simulink model "D_framewiseincremental_simple_vs_cascaded"  (R2017a)
settings: Solver=ode45  StartTime=0.0  StopTime=200  FixedStep=0.05  RelTol=1e-3  EnableMultiTasking=on
values from neighbouring files (symbols this model uses):
  B = [1 0.5 -0.5 -1 0 0.5 ; 0 0 0 0 2 0 ; -0.05 -0.02 0.02 0.05 0 2 ; -1 -1 -1 -1 -2 0]    [A_runSimulation.m]    (also in C_runSimulation.m; D_runSimulation.m; E_runSimulation.m; F_runSimulation.m)
  gain_four = rand()*2    [A_runSimulation.m]    (also in C_runSimulation.m = 0; D_runSimulation.m; E_runSimulation.m = 0; F_runSimulation.m = 0)
  gain_one = rand()*2    [A_runSimulation.m]    (also in C_runSimulation.m = 0; D_runSimulation.m; E_runSimulation.m = 0; F_runSimulation.m = 0)
  gain_three = rand()*2    [A_runSimulation.m]    (also in C_runSimulation.m = 0; D_runSimulation.m; E_runSimulation.m = 0; F_runSimulation.m = 0)
  gain_two = rand()*2    [A_runSimulation.m]    (also in C_runSimulation.m = 0; D_runSimulation.m; E_runSimulation.m = 0; F_runSimulation.m = 0)
  reduction_type = 1    [A_runSimulation.m]    (also in C_runSimulation.m = 2; D_runSimulation.m; E_runSimulation.m = 2)
  seed_four = k + 30    [A_runSimulation.m]    (also in C_runSimulation.m; D_runSimulation.m; E_runSimulation.m; F_runSimulation.m)
  seed_one = k    [A_runSimulation.m]    (also in C_runSimulation.m; D_runSimulation.m; E_runSimulation.m; F_runSimulation.m)
  seed_three = k + 20    [A_runSimulation.m]    (also in C_runSimulation.m; D_runSimulation.m; E_runSimulation.m; F_runSimulation.m)
  seed_two = k + 10    [A_runSimulation.m]    (also in C_runSimulation.m; D_runSimulation.m; E_runSimulation.m; F_runSimulation.m)
  signal_gain = j    [A_runSimulation.m]    (also in C_runSimulation.m; D_runSimulation.m; E_runSimulation.m = 0.3; F_runSimulation.m)
  simulate_envelope = 1    [A_runSimulation.m]    (also in C_runSimulation.m = 0; D_runSimulation.m; E_runSimulation.m = 0)
  u_lim = [[-0.5 -0.5 -0.5 -0.5 -0.5 -0.5]' [0.5 0.5 0.5 0.5 0.5 0.5]']    [A_runSimulation.m]    (also in C_runSimulation.m; D_runSimulation.m; E_runSimulation.m; F_runSimulation.m)
  udot_lim = [[2 2 2 2 2 2]']    [A_runSimulation.m]    (also in C_runSimulation.m; D_runSimulation.m; E_runSimulation.m; F_runSimulation.m)
  W = eye(6)    [A_runSimulation.m]    (also in C_runSimulation.m; D_runSimulation.m; E_runSimulation.m; F_runSimulation.m)
libraries: dspsrcs4 x8
settings Model: Creator=markvoskuijl  LastModifiedBy=Luca
settings DataIOCC: LimitDataPoints=on  SaveFormat=Array  SignalLoggingSaveFormat=ModelDataLogs
settings OptimizationCC: ExpressionDepthLimit=2147483647  LifeSpan=inf
settings DebuggingCC: UnderspecifiedInitializationDetection=Classic  MergeDetectMultiDrivingBlocksExec=none  SolverPrmCheckMsg=warning  FcnCallInpInsideContextMsg=warning  StateNameClashWarn=warning  SFUnexpectedBacktrackingDiag=warning  SFNoUnconditionalDefaultTransitionDiag=warning  SFExecutionAtInitializationDiag=none
settings HardwareCC: ProdBitPerPointer=32  ProdBitPerSizeT=32  ProdBitPerPtrDiffT=32  ProdLargestAtomicFloat=None  ProdIntDivRoundTo=Undefined  ProdEndianess=Unspecified  ProdWordSize=32  ProdHWDeviceType=32-bit Generic
settings ModelReferenceCC: PropagateSignalLabelsOutOfModel=off
settings GRTTargetCC: TargetLangStandard=C89/C90 (ANSI)  GeneratePreprocessorConditionals=Disable all  CombineOutputUpdateFcns=off  GRTInterface=on
settings ConfigComp: CovMetricSettings=dw  CovHtmlReporting=on  CovSaveCumulativeToWorkspaceVar=on  CovSaveSingleToWorkspaceVar=on  CovExternalEMLEnable=off

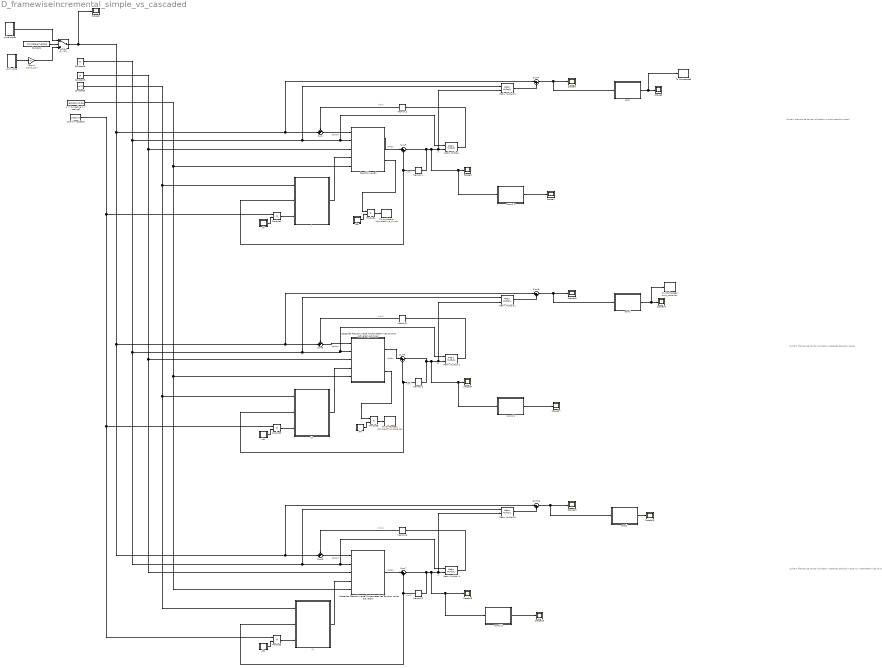
== system D_framewiseincremental_simple_vs_cascaded ==
  note: deltam
  note: deltau
  note: ut
  note: u(t-1)
  note: m(t-1)
  note: durham
      | (framewise control allocation
      | simple pseudoinverse)
  note: deltam
  note: u(t-1)
  note: m(t-1)
  note: ut
  note: durham
      | (framewise control allocation
      | cascaded pseudoinverse
      | no underdetermined solution)
  note: deltau
  note: m(t-1)
  note: deltam
  note: u(t-1)
  note: ut
  note: deltau
  note: durham
      | (framewise control allocation
      | cascaded pseudoinverse)
  "1 -> truncating 2 -> scaling1" : Constant  Value=reduction_type
  Cascaded Pseudoinverse (Under deterined solution never activated) : MATLAB Function  TreatAsAtomicUnit=on
  Cascaded Pseudoinverse (Under determined solution activated just once) : MATLAB Function  TreatAsAtomicUnit=on
  Constant : Constant  Value=simulate_envelope
  Constant4 : Constant  Value=u_lim
  Constant5 : Constant  Value=W
  Constant6 : Constant  Value=B
  Gain4 : Gain  Gain=signal_gain
  I : MATLAB Function  TreatAsAtomicUnit=on
  I1 : MATLAB Function  TreatAsAtomicUnit=on
  I3 : MATLAB Function  TreatAsAtomicUnit=on
  Matrix Multiply{,1..5} (6 alike) : Product  Multiplication=Matrix(*)
  Memory{1..6} (6 alike) : Memory
  Product{1..5} (5 alike) : Product
  Pseudoinverse1 : MATLAB Function  TreatAsAtomicUnit=on
  Scope{1..3,5..6,13..15,19,24..27} (13 alike) : Scope
  Sum : Sum  Inputs=-+|
  Sum10 : Sum  Inputs=|-+
  Sum3 : Sum  Inputs=|++
  Sum4 : Sum  Inputs=|-+
  Sum5 : Sum  Inputs=-+|
  Sum6 : Sum  Inputs=-+|
  Sum7 : Sum  Inputs=|++
  Sum8 : Sum  Inputs=|++
  Sum9 : Sum  Inputs=|-+
  Switch : Switch  Threshold=1
  To Workspace : ToWorkspace  VariableName=saturatedtime_simple  SampleTime=-1
      settings: Save2DSignal=2-D array (concatenate along first dimension)
  To Workspace1 : ToWorkspace  VariableName=saturatedtime_cascaded  SampleTime=-1
      settings: Save2DSignal=2-D array (concatenate along first dimension)
  To Workspace2 : ToWorkspace  VariableName=error_cascaded  SampleTime=-1
      settings: Save2DSignal=2-D array (concatenate along first dimension)
  To Workspace3 : ToWorkspace  VariableName=error_simple  SampleTime=-1
      settings: Save2DSignal=2-D array (concatenate along first dimension)
  dt : Subsystem
  dt1 : Subsystem
  dt2 : Subsystem
  dt3 : Subsystem
  dt4 : Subsystem
  error : MATLAB Function  TreatAsAtomicUnit=on
  error1 : MATLAB Function  TreatAsAtomicUnit=on
  error2 : MATLAB Function  TreatAsAtomicUnit=on
  norm2 1 : MATLAB Function  TreatAsAtomicUnit=on
  norm2 2 : MATLAB Function  TreatAsAtomicUnit=on
  norm2 3 : MATLAB Function  TreatAsAtomicUnit=on
  pink noise : Subsystem
  udot lim rad/sec3 : Constant  Value=udot_lim
  white noise : Subsystem
  wires:
  Sum/1 -> Pseudoinverse1/1(m)
  Matrix Multiply/1 -> Memory2/1
  I/1(I) -> Pseudoinverse1/4(u_lim)
  Pseudoinverse1/1(u) -> Sum3/1
  Product1/1 -> I/3(udotdt_lim)  "udot dt"
  dt/1(dt) -> Product1/2
  Memory1/1 -> I/2(u), Sum3/2
  Memory2/1 -> Sum/1
  Matrix Multiply3/1 -> Sum4/2
  Sum4/1 -> error/1(e), Scope6/1
  Sum3/1 -> norm2 1/1(u), Scope5/1, Matrix Multiply3/2, Matrix Multiply/2, Memory1/1
  Matrix Multiply2/1 -> Sum9/2
  Sum8/1 -> norm2 2/1(u), Scope14/1, Matrix Multiply2/2, Matrix Multiply1/2, Memory3/1
  dt1/1(dt) -> Product2/2
  Memory4/1 -> Sum5/1
  Sum9/1 -> error1/1(e), Scope15/1
  Memory3/1 -> I3/2(u), Sum8/2
  Matrix Multiply1/1 -> Memory4/1
  Product2/1 -> I3/3(udotdt_lim)  "udot dt"
  Cascaded Pseudoinverse (Under determined solution activated just once)/1(u) -> Sum8/1
  Sum5/1 -> Cascaded Pseudoinverse (Under determined solution activated just once)/1(m)
  I3/1(I) -> Cascaded Pseudoinverse (Under determined solution activated just once)/4(u_lim)
  Cascaded Pseudoinverse (Under deterined solution never activated)/1(u) -> Sum7/1
  Sum6/1 -> Cascaded Pseudoinverse (Under deterined solution never activated)/1(m)
  Constant4/1 -> I/1(u_lim), I1/1(u_lim), I3/1(u_lim)
  dt2/1(dt) -> Product3/2
  Product3/1 -> I1/3(udotdt_lim)  "udot dt"
  Memory5/1 -> I1/2(u), Sum7/2
  Constant6/1 -> Matrix Multiply3/1, Matrix Multiply/1, Pseudoinverse1/2(B), Matrix Multiply5/1, Cascaded Pseudoinverse (Under deterined solution never activated)/2(B), Matrix Multiply4/1, Matrix Multiply2/1, Cascaded Pseudoinverse (Under determined solution activated just once)/2(B), Matrix Multiply1/1
  Matrix Multiply4/1 -> Memory6/1
  Constant5/1 -> Cascaded Pseudoinverse (Under deterined solution never activated)/3(W), Cascaded Pseudoinverse (Under determined solution activated just once)/3(W), Pseudoinverse1/3(W)
  Memory6/1 -> Sum6/1
  udot lim rad/sec3/1 -> Product2/1, Product3/1, Product1/1
  "1 -> truncating 2 -> scaling1"/1 -> Pseudoinverse1/5(reductionType), Cascaded Pseudoinverse (Under deterined solution never activated)/5(reductionType), Cascaded Pseudoinverse (Under determined solution activated just once)/5(reductionType)
  Matrix Multiply5/1 -> Sum10/2
  I1/1(I) -> Cascaded Pseudoinverse (Under deterined solution never activated)/4(u_lim)
  error1/1(error) -> To Workspace2/1, Scope24/1
  Sum10/1 -> error2/1(e), Scope19/1
  Sum7/1 -> norm2 3/1(u), Scope13/1, Matrix Multiply5/2, Matrix Multiply4/2, Memory5/1
  Switch/1 -> Scope3/1, Sum4/1, Sum/2, Sum10/1, Sum6/2, Sum9/1, Sum5/2
  error/1(error) -> To Workspace3/1, Scope2/1
  error2/1(error) -> Scope25/1
  norm2 1/1(norm2) -> Scope1/1
  norm2 2/1(norm2) -> Scope27/1
  norm2 3/1(norm2) -> Scope26/1
  pink noise/1(Out1) -> Gain4/1
  Gain4/1 -> Switch/3
  Constant/1 -> Switch/2
  white noise/1(Out1) -> Switch/1
  Pseudoinverse1/2(saturated) -> Product4/1
  dt3/1(dt) -> Product4/2
  Product4/1 -> To Workspace/1
  Cascaded Pseudoinverse (Under determined solution activated just once)/2(saturated) -> Product5/1
  dt4/1(dt) -> Product5/2
  Product5/1 -> To Workspace1/1

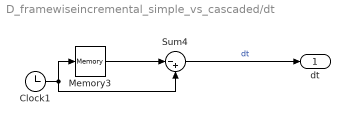
== system D_framewiseincremental_simple_vs_cascaded/dt ==
  Clock1 : Clock
  Memory3 : Memory
  Sum4 : Sum  Inputs=|-+
  dt : Outport
  wires:
  Clock1/1 -> Sum4/2, Memory3/1
  Memory3/1 -> Sum4/1
  Sum4/1 -> dt/1  "dt"

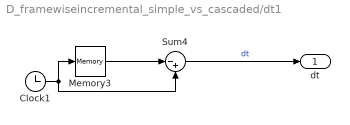
== system D_framewiseincremental_simple_vs_cascaded/dt1 ==
  Clock1 : Clock
  Memory3 : Memory
  Sum4 : Sum  Inputs=|-+
  dt : Outport
  wires:
  Clock1/1 -> Sum4/2, Memory3/1
  Memory3/1 -> Sum4/1
  Sum4/1 -> dt/1  "dt"

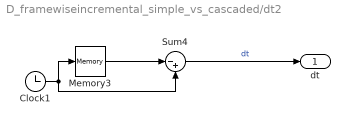
== system D_framewiseincremental_simple_vs_cascaded/dt2 ==
  Clock1 : Clock
  Memory3 : Memory
  Sum4 : Sum  Inputs=|-+
  dt : Outport
  wires:
  Clock1/1 -> Sum4/2, Memory3/1
  Memory3/1 -> Sum4/1
  Sum4/1 -> dt/1  "dt"

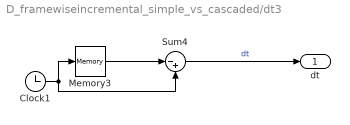
== system D_framewiseincremental_simple_vs_cascaded/dt3 ==
  Clock1 : Clock
  Memory3 : Memory
  Sum4 : Sum  Inputs=|-+
  dt : Outport
  wires:
  Clock1/1 -> Sum4/2, Memory3/1
  Memory3/1 -> Sum4/1
  Sum4/1 -> dt/1  "dt"

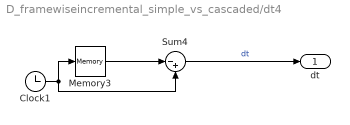
== system D_framewiseincremental_simple_vs_cascaded/dt4 ==
  Clock1 : Clock
  Memory3 : Memory
  Sum4 : Sum  Inputs=|-+
  dt : Outport
  wires:
  Clock1/1 -> Sum4/2, Memory3/1
  Memory3/1 -> Sum4/1
  Sum4/1 -> dt/1  "dt"

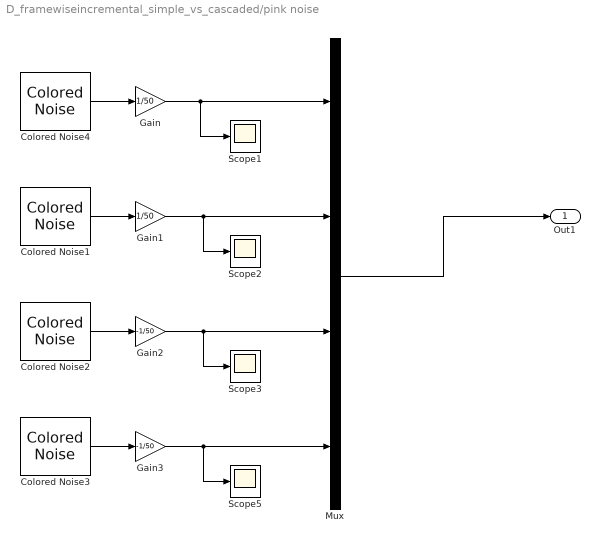
== system D_framewiseincremental_simple_vs_cascaded/pink noise ==
  Colored Noise1 : dspsrcs4/Colored Noise  Color=custom  InverseFrequencyPower=2  NumChannels=1  OutputDataType=single  SamplesPerFrame=1  SampleTime=0.1  RandomStream=mt19937ar with seed  Seed=seed_two  SimulateUsing=Interpreted execution
      settings: SourceProductName=DSP System Toolbox  SourceProductBaseCode=DS
  Colored Noise2 : dspsrcs4/Colored Noise  Color=custom  InverseFrequencyPower=2  NumChannels=1  OutputDataType=single  SamplesPerFrame=1  SampleTime=0.1  RandomStream=mt19937ar with seed  Seed=seed_three  SimulateUsing=Interpreted execution
      settings: SourceProductName=DSP System Toolbox  SourceProductBaseCode=DS
  Colored Noise3 : dspsrcs4/Colored Noise  Color=custom  InverseFrequencyPower=2  NumChannels=1  OutputDataType=single  SamplesPerFrame=1  SampleTime=0.1  RandomStream=mt19937ar with seed  Seed=seed_four  SimulateUsing=Interpreted execution
      settings: SourceProductName=DSP System Toolbox  SourceProductBaseCode=DS
  Colored Noise4 : dspsrcs4/Colored Noise  Color=custom  InverseFrequencyPower=2  NumChannels=1  OutputDataType=single  SamplesPerFrame=1  SampleTime=0.1  RandomStream=mt19937ar with seed  Seed=seed_one  SimulateUsing=Interpreted execution
      settings: SourceProductName=DSP System Toolbox  SourceProductBaseCode=DS
  Gain : Gain  Gain=1/50
  Gain1 : Gain  Gain=1/50
  Gain2 : Gain  Gain=-1/50
  Gain3 : Gain  Gain=-1/50
  Mux : Mux
  Scope{1..3,5} (4 alike) : Scope
  Out1 : Outport
  wires:
  Colored Noise4/1 -> Gain/1
  Colored Noise1/1 -> Gain1/1
  Colored Noise2/1 -> Gain2/1
  Gain/1 -> Scope1/1, Mux/1
  Gain1/1 -> Scope2/1, Mux/2
  Gain2/1 -> Scope3/1, Mux/3
  Mux/1 -> Out1/1
  Gain3/1 -> Mux/4, Scope5/1
  Colored Noise3/1 -> Gain3/1

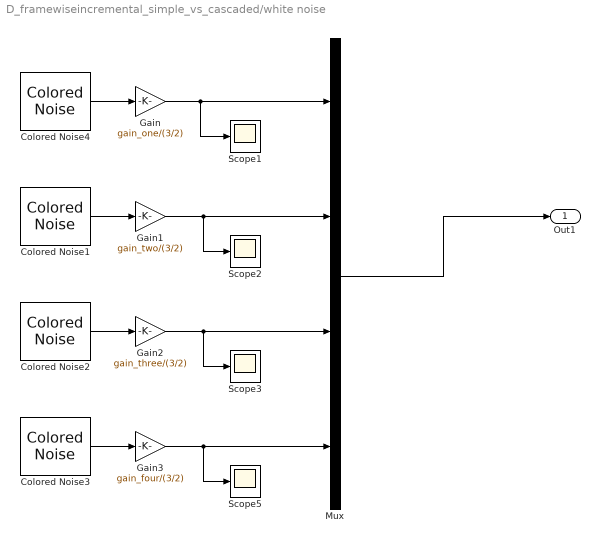
== system D_framewiseincremental_simple_vs_cascaded/white noise ==
  Colored Noise1 : dspsrcs4/Colored Noise  Color=white  InverseFrequencyPower=2  NumChannels=1  OutputDataType=single  SamplesPerFrame=1  SampleTime=0.1  RandomStream=mt19937ar with seed  Seed=seed_two  SimulateUsing=Interpreted execution
      settings: SourceProductName=DSP System Toolbox  SourceProductBaseCode=DS
  Colored Noise2 : dspsrcs4/Colored Noise  Color=white  InverseFrequencyPower=2  NumChannels=1  OutputDataType=single  SamplesPerFrame=1  SampleTime=0.1  RandomStream=mt19937ar with seed  Seed=seed_three  SimulateUsing=Interpreted execution
      settings: SourceProductName=DSP System Toolbox  SourceProductBaseCode=DS
  Colored Noise3 : dspsrcs4/Colored Noise  Color=white  InverseFrequencyPower=2  NumChannels=1  OutputDataType=single  SamplesPerFrame=1  SampleTime=0.1  RandomStream=mt19937ar with seed  Seed=seed_four  SimulateUsing=Interpreted execution
      settings: SourceProductName=DSP System Toolbox  SourceProductBaseCode=DS
  Colored Noise4 : dspsrcs4/Colored Noise  Color=white  InverseFrequencyPower=2  NumChannels=1  OutputDataType=single  SamplesPerFrame=1  SampleTime=0.1  RandomStream=mt19937ar with seed  Seed=seed_one  SimulateUsing=Interpreted execution
      settings: SourceProductName=DSP System Toolbox  SourceProductBaseCode=DS
  Gain : Gain  Gain=gain_one/(3/2)
  Gain1 : Gain  Gain=gain_two/(3/2)
  Gain2 : Gain  Gain=gain_three/(3/2)
  Gain3 : Gain  Gain=gain_four/(3/2)
  Mux : Mux
  Scope{1..3,5} (4 alike) : Scope
  Out1 : Outport
  wires:
  Colored Noise4/1 -> Gain/1
  Colored Noise1/1 -> Gain1/1
  Colored Noise2/1 -> Gain2/1
  Gain/1 -> Scope1/1, Mux/1
  Gain1/1 -> Scope2/1, Mux/2
  Gain2/1 -> Scope3/1, Mux/3
  Mux/1 -> Out1/1
  Gain3/1 -> Mux/4, Scope5/1
  Colored Noise3/1 -> Gain3/1

== matlab function D_framewiseincremental_simple_vs_cascaded/Pseudoinverse1 ==
  data: m input; u output; B input; W input; u_lim input; reductionType input; saturated output
function [u, saturated] = Pseudoinverse(m, B, W, u_lim, reductionType)
coder.varsize('u_index', 'Br', 'Wr', 'u_sat');

%check if the matrices are correct
    if not(isequal(size(u_lim,1),size(B,2),size(W,1),size(W,2))...
       && isequal(length(m),size(B,1)))
        error ('input matrix dimensions do not match')
    end
    
%assign to every equation an index    
    u_index = [1:length(u_lim)].';
    
%check the type of system and then compute the pseudoinverse 1st step
    order = size(B,2)-size(B,1);

    if order > 0 %over-determined, solution that minimizes the 2norm
        u = inv(W)*B'*inv(B*inv(W)*B')*m;
    elseif order < 0 %under-determined, solution that minimizes the error
        u = inv(B'*B)*B'*m;   
    else %order = 0, sqared thus invertiBrle
        u = inv(B)*m;
    end

%deifne u_sat vector
    u_sat = zeros(length(u),1);
    
    saturated = 0;
    
%check if the first iteration solution is correct then return    
    if not(any(u < u_lim(:,1))||any(u > u_lim(:,2)))  
        return
    end
    
    saturated = 1; 
    
%The software continues only if the solution has to be reduced
%reduce their value
    switch reductionType
        case 1 %truncation
            %takes note of which one are out of their bounds
                u_sat(u < u_lim(:,1)) = 1;
                u_sat(u > u_lim(:,2)) = 1;
                
            %trucate
                u = min(u, u_lim(:,2));
                u = max(u, u_lim(:,1));

        case 2 %scaling solution -> direction preserving
            %reduce
                a = zeros(length(u),1);

                for i = 1:length(u)
                    if u(i)>0
                       a(i) = abs(u(i)/u_lim(i,2));
                    elseif u(i)<0
                       a(i) = abs(u(i)/u_lim(i,1));
                    else
                       a(i) = 0; 
                    end          
                end
                a_max = max(a);
                u = u/a_max;
            
            %takes note of which one are out of their bounds
                u_sat(u == u_lim(:,2)) = 1;
                u_sat(u == u_lim(:,1)) = 1;
            
    end
    
return
    
end

== matlab function D_framewiseincremental_simple_vs_cascaded/I1 ==
  data: u_lim input; u input; udotdt_lim input; I output
function I = computeIntersection(u_lim, u, udotdt_lim)
%check if the matrices are correct
    if not(isequal(size(u_lim,1),size(udotdt_lim,1), size(u,1)))
        error ('input matrix dimensions do not match')
    end

%declare space of intersection
    I = zeros(length(u_lim),2);
    
    I(:,1) = -min(udotdt_lim, abs(u_lim(:,1)-u));
    I(:,2) = min(+udotdt_lim, abs(u_lim(:,2)-u));
    
end

== matlab function D_framewiseincremental_simple_vs_cascaded/norm2 1 ==
  data: u input; norm2 output
function norm2 = norm2(u)

    norm2 = sum(u.^2);

end

== matlab function D_framewiseincremental_simple_vs_cascaded/I ==
  data: u_lim input; u input; udotdt_lim input; I output
function I = computeIntersection(u_lim, u, udotdt_lim)
%check if the matrices are correct
    if not(isequal(size(u_lim,1),size(udotdt_lim,1), size(u,1)))
        error ('input matrix dimensions do not match')
    end

%declare space of intersection
    I = zeros(length(u_lim),2);
    
    I(:,1) = -min(udotdt_lim, abs(u_lim(:,1)-u));
    I(:,2) = min(+udotdt_lim, u_lim(:,2)-u);
    
end

== matlab function D_framewiseincremental_simple_vs_cascaded/Cascaded Pseudoinverse (Under deterined solution never activated) ==
  data: m input; u output; B input; W input; u_lim input; reductionType input
function u = CascadedPseudoinverse(m, B, W, u_lim, reductionType)
coder.varsize('u_index', 'Br', 'Wr', 'u_sat');

%check if the matrices are correct
    if not(isequal(size(u_lim,1),size(B,2),size(W,1),size(W,2))...
       && isequal(length(m),size(B,1)))
        error ('input matrix dimensions do not match')
    end
    
%assign to every equation an index    
    u_index = [1:length(u_lim)].';
    
%check the type of system and then compute the pseudoinverse 1st step
    order = size(B,2)-size(B,1);

    if order > 0 %over-determined, solution that minimizes the 2norm
        u = inv(W)*B'*inv(B*inv(W)*B')*m;
    elseif order < 0 %under-determined, solution that minimizes the error
        u = inv(B'*B)*B'*m;   
    else %order = 0, sqared thus invertiBrle
        u = inv(B)*m;
    end

%deifne u_sat vector
    u_sat = zeros(length(u),1);
    
%check if the first iteration solution is correct then return    
    if not(any(u < u_lim(:,1))||any(u > u_lim(:,2)))  
        return
    end
    
%The software continues only if the solution has to be reduced
%reduce their value
    switch reductionType
        case 1 %truncation
            %takes note of which one are out of their bounds
                u_sat(u < u_lim(:,1)) = 1;
                u_sat(u > u_lim(:,2)) = 1;
                
            %trucate
                u = min(u, u_lim(:,2));
                u = max(u, u_lim(:,1));

        case 2 %scaling solution -> direction preserving
            %reduce
                a = zeros(length(u),1);

                for i = 1:length(u)
                    if u(i)>0
                       a(i) = abs(u(i)/u_lim(i,2));
                    elseif u(i)<0
                       a(i) = abs(u(i)/u_lim(i,1));
                    else
                       a(i) = 0; 
                    end          
                end
                a_max = max(a);
                u = u/a_max;
            
            %takes note of which one are out of their bounds
                u_sat(u == u_lim(:,2)) = 1;
                u_sat(u == u_lim(:,1)) = 1;
            
    end

    
%Recursively compute until solution is found or all the effectors are saturated
    Br = B;
    Wr = W;
    cycleAgain = 1;

    while(cycleAgain == 1) %till we run out of effectors
        %compute the residual moment
            m_res = m - B*u;
            
        %reduce the system 
            u_index(u_sat == 1)= [];
                if isempty(u_index)
                    return
                end
                
            Br(:,u_sat == 1)=[];
            Wr(:,u_sat == 1)=[]; Wr(u_sat == 1,:)=[];
        
        %check the type of system and then compute the pseudoinverse
            order = size(Br,2)-size(Br,1);

            if order > 0 %over-determined, solution that minimizes the 2norm
                ur = inv(Wr)*Br.'*inv(Br*inv(Wr)*Br.')*m_res;
            elseif order < 0 %under-determined, solution that minimizes the error
                return %never solve underdetermined solution
            else %order = 0, sqared thus invertiBrle
                ur = inv(Br)*m_res;
                cycleAgain = 0;
            end
            
        %sum the freshly new result with the pre existing u
            ut = u;
            ut(u_index,1) = u(u_index,1) + ur;

        %reduce the solution, if needed. If not needed exit the cycle
            if not(any(ut < u_lim(:,1))||any(ut > u_lim(:,2))) %Wre found a solution then Brreak
                u = ut;
                return 
                
            else %some deflectors are past their limit                    
                %reduce their value
                    switch reductionType
                        case 1 %truncation
                            %takes note of which one are out of their bounds
                                u_sat = zeros(length(ur),1);
                                u_sat(ut(u_index) < u_lim(u_index,1)) = 1;
                                u_sat(ut(u_index) > u_lim(u_index,2)) = 1;
                            
                            %truncate
                                u(u_index) = min(ut(u_index), u_lim(u_index,2));
                                u(u_index) = max(u(u_index), u_lim(u_index,1));

                        case 2 %scaling solution -> direction preserving
                                a = zeros(length(u_index),1);

                                for i = 1:length(u_index)
                                    if ur(i)>0
                                       a(i) = abs(ur(i)/(u_lim(u_index(i),2)-u(u_index(i))));
                                    elseif ur(i)<0
                                       a(i) = abs(ur(i)/(u_lim(u_index(i),1)-u(u_index(i))));
                                    else
                                       a(i) = 0; 
                                    end          
                                end
                                a_max = max(a);
                                ur = ur/a_max; 
                            
                            %takes note of which one are out of their bounds
                                u_sat = zeros(length(ur),1);
                                u_sat(a == a_max) = 1;
                            
                            %sum the freshly new result with the pre existing u
                                u(u_index,1) = u(u_index,1) + ur;
                    end
            end
    end

    
end

== matlab function D_framewiseincremental_simple_vs_cascaded/error1 ==
  data: e input; error output
function error = error(e)

    error = sum(abs(e));

end

== matlab function D_framewiseincremental_simple_vs_cascaded/error ==
  data: e input; error output
function error = error(e)

    error = sum(abs(e));

end

== matlab function D_framewiseincremental_simple_vs_cascaded/norm2 2 ==
  data: u input; norm2 output
function norm2 = norm2(u)

    norm2 = sum(u.^2);

end

== matlab function D_framewiseincremental_simple_vs_cascaded/Cascaded Pseudoinverse (Under determined solution activated just once) ==
  data: m input; u output; B input; W input; u_lim input; reductionType input; saturated output
function [u , saturated] = CascadedPseudoinverse(m, B, W, u_lim, reductionType)
coder.varsize('u_index', 'Br', 'Wr', 'u_sat');

%check if the matrices are correct
    if not(isequal(size(u_lim,1),size(B,2),size(W,1),size(W,2))...
       && isequal(length(m),size(B,1)))
        error ('input matrix dimensions do not match')
    end
    
%assign to every equation an index    
    u_index = [1:length(u_lim)].';
    
%check the type of system and then compute the pseudoinverse 1st step
    order = size(B,2)-size(B,1);

    if order > 0 %over-determined, solution that minimizes the 2norm
        u = inv(W)*B'*inv(B*inv(W)*B')*m;
    elseif order < 0 %under-determined, solution that minimizes the error
        u = inv(B'*B)*B'*m;   
    else %order = 0, sqared thus invertiBrle
        u = inv(B)*m;
    end

%deifne u_sat vector
    u_sat = zeros(length(u),1);
    
    saturated = 0;
    
%check if the first iteration solution is correct then return    
    if not(any(u < u_lim(:,1))||any(u > u_lim(:,2)))  
        return
    end
    
    saturated = 1;
    
%The software continues only if the solution has to be reduced
%reduce their value
    switch reductionType
        case 1 %truncation
            %takes note of which one are out of their bounds
                u_sat(u < u_lim(:,1)) = 1;
                u_sat(u > u_lim(:,2)) = 1;
                
            %trucate
                u = min(u, u_lim(:,2));
                u = max(u, u_lim(:,1));

        case 2 %scaling solution -> direction preserving
            %reduce
                a = zeros(length(u),1);

                for i = 1:length(u)
                    if u(i)>0
                       a(i) = abs(u(i)/u_lim(i,2));
                    elseif u(i)<0
                       a(i) = abs(u(i)/u_lim(i,1));
                    else
                       a(i) = 0; 
                    end          
                end
                a_max = max(a);
                u = u/a_max;
            
            %takes note of which one are out of their bounds
                u_sat(u == u_lim(:,2)) = 1;
                u_sat(u == u_lim(:,1)) = 1;
            
    end

    
%Recursively compute until solution is found or all the effectors are saturated
    Br = B;
    Wr = W;
    cycleAgain = 1

    while(cycleAgain == 1) %till we run out of effectors
        %compute the residual moment
            m_res = m - B*u;
            
        %reduce the system 
            u_index(u_sat == 1)= [];
                if isempty(u_index)
                    return
                end
                
            Br(:,u_sat == 1)=[];
            Wr(:,u_sat == 1)=[]; Wr(u_sat == 1,:)=[];
        
        %check the type of system and then compute the pseudoinverse
            order = size(Br,2)-size(Br,1);

            if order > 0 %over-determined, solution that minimizes the 2norm
                ur = inv(Wr)*Br.'*inv(Br*inv(Wr)*Br.')*m_res;
            elseif order < 0 %under-determined, solution that minimizes the error
                ur = inv(Br'*Br)*Br'*m_res;  
                cycleAgain = 0; %only one underdetermined solution is allowed
            else %order = 0, sqared thus invertiBrle
                ur = inv(Br)*m_res;
            end
            
        %sum the freshly new result with the pre existing u
            ut = u;
            ut(u_index,1) = u(u_index,1) + ur;

        %reduce the solution, if needed. If not needed exit the cycle
            if not(any(ut < u_lim(:,1))||any(ut > u_lim(:,2))) %Wre found a solution then Brreak
                u = ut;
                return 
                
            else %some deflectors are past their limit                    
                %reduce their value
                    switch reductionType
                        case 1 %truncation
                            %takes note of which one are out of their bounds
                                u_sat = zeros(length(ur),1);
                                u_sat(ut(u_index) < u_lim(u_index,1)) = 1;
                                u_sat(ut(u_index) > u_lim(u_index,2)) = 1;
                            
                            %truncate
                                u(u_index) = min(ut(u_index), u_lim(u_index,2));
                                u(u_index) = max(u(u_index), u_lim(u_index,1));

                        case 2 %scaling solution -> direction preserving
                                a = zeros(length(u_index),1);

                                for i = 1:length(u_index)
                                    if ur(i)>0
                                       a(i) = abs(ur(i)/(u_lim(u_index(i),2)-u(u_index(i))));
                                    elseif ur(i)<0
                                       a(i) = abs(ur(i)/(u_lim(u_index(i),1)-u(u_index(i))));
                                    else
                                       a(i) = 0; 
                                    end          
                                end
                                a_max = max(a);
                                ur = ur/a_max; 
                            
                            %takes note of which one are out of their bounds
                                u_sat = zeros(length(ur),1);
                                u_sat(a == a_max) = 1;
                            
                            %sum the freshly new result with the pre existing u
                                u(u_index,1) = u(u_index,1) + ur;
                    end
            end
    end

    
end

== matlab function D_framewiseincremental_simple_vs_cascaded/error2 ==
  data: e input; error output
function error = error(e)

    error = sum(abs(e));

end

== matlab function D_framewiseincremental_simple_vs_cascaded/norm2 3 ==
  data: u input; norm2 output
function norm2 = norm2(u)

    norm2 = sum(u.^2);

end

== matlab function D_framewiseincremental_simple_vs_cascaded/I3 ==
  data: u_lim input; u input; udotdt_lim input; I output
function I = computeIntersection(u_lim, u, udotdt_lim)
%check if the matrices are correct
    if not(isequal(size(u_lim,1),size(udotdt_lim,1), size(u,1)))
        error ('input matrix dimensions do not match')
    end

%declare space of intersection
    I = zeros(length(u_lim),2);
    
    I(:,1) = -min(udotdt_lim, abs(u_lim(:,1)-u));
    I(:,2) = min(+udotdt_lim, abs(u_lim(:,2)-u));
    
end
